simulink model "ROB599_HW4_P5"  (R2023b)
settings: Solver=VariableStepAuto  StartTime=0.0  StopTime=10.0  RelTol=1e-3
undefined symbols (not defined in the file or in its folder): param
settings Model: Creator=anatoliikalinin  LastModifiedBy=anatoliikalinin

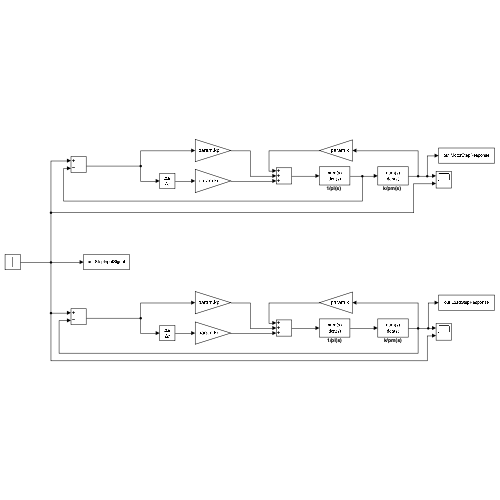
[thumbnail: Simulink's stored preview of the top-level diagram]
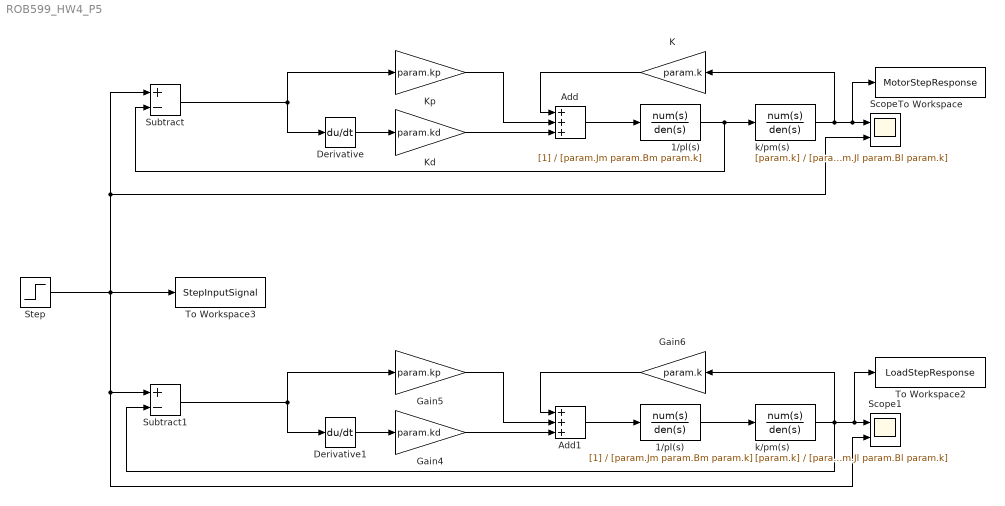
== system ROB599_HW4_P5 ==
  1/pl(s) : TransferFcn  Denominator=[param.Jm param.Bm param.k]
  "1/pl(s) " : TransferFcn  Denominator=[param.Jm param.Bm param.k]
  Add : Sum  Inputs=+++
  Add1 : Sum  Inputs=+++
  Derivative : Derivative
  Derivative1 : Derivative
  Gain4 : Gain  Gain=param.kd
  Gain5 : Gain  Gain=param.kp
  Gain6 : Gain  Gain=param.k
  K : Gain  Gain=param.k
  Kd : Gain  Gain=param.kd
  Kp : Gain  Gain=param.kp
  Scope : Scope  NumInputPorts=2
  Scope1 : Scope  NumInputPorts=2
  Step : Step  SampleTime=0
  Subtract : Sum  Inputs=+-
  Subtract1 : Sum  Inputs=+-
  To Workspace : ToWorkspace  VariableName=MotorStepResponse  SaveFormat=Timeseries  SampleTime=-1
  To Workspace2 : ToWorkspace  VariableName=LoadStepResponse  SaveFormat=Timeseries  SampleTime=-1
  To Workspace3 : ToWorkspace  VariableName=StepInputSignal  SaveFormat=Timeseries  SampleTime=-1
  k/pm(s) : TransferFcn  Numerator=[param.k]  Denominator=[param.Jl param.Bl param.k]
  "k/pm(s) " : TransferFcn  Numerator=[param.k]  Denominator=[param.Jl param.Bl param.k]
  wires:
  Derivative/1 -> Kd/1
  Kp/1 -> Add/2
  Kd/1 -> Add/3
  Add/1 -> "1/pl(s) "/1
  "1/pl(s) "/1 -> Subtract/2, "k/pm(s) "/1
  "k/pm(s) "/1 -> K/1, To Workspace/1, Scope/1
  Step/1 -> To Workspace3/1, Scope1/2, Subtract1/1, Subtract/1, Scope/2
  Subtract/1 -> Kp/1, Derivative/1
  K/1 -> Add/1
  Gain6/1 -> Add1/1
  Subtract1/1 -> Derivative1/1, Gain5/1
  k/pm(s)/1 -> Subtract1/2, To Workspace2/1, Scope1/1, Gain6/1
  Add1/1 -> 1/pl(s)/1
  Gain4/1 -> Add1/3
  Gain5/1 -> Add1/2
  Derivative1/1 -> Gain4/1
  1/pl(s)/1 -> k/pm(s)/1
